simulink model "Urban_Air_Mobility_v3"  (R2021a)
settings: Solver=ode4  StartTime=0.0  StopTime=50  FixedStep=0.01  RelTol=1e-3
model workspace (MAT data in the model file):
  op_trim2 : handle (value not decoded)
undefined symbols (not defined in the file or in its folder): BackProp, Earth, ForwProp, geo, initialise, mass, simsetup, WGS84
libraries: dspindex x6, aerolibactuator x4, sharedutil x3, simulink x3, aerolibasang x2, aerolibtransform2 x2, aerolibutil x2, shared6dof x1, aerolibatmos2 x1, sharedtransform x1, aerolibconvert2 x1
(part 3 of 3)

== system Urban_Air_Mobility_v3/Urban Air Vehicle Airframe Flight Dynamic Model/Landing_gear_Model/Landing Gear (with steer 4)/Main_gear_right_friction_forces/Velocity at MGR in ground path ==
  DCM_B_to_E : Inport
  V_b : Inport  Port=2
  "[p, q, r]" : Inport  Port=3
  P_gear : Inport  Port=4
  P_cg : Inport  Port=5
  Euler : Inport  Port=6
  Demux : Demux  Outputs=3
  Ground Path Velocities : Subsystem
  Matrix Multiply1 : Product  Multiplication=Matrix(*)
  Mux2 : Mux  Inputs=3
  Velocity at gear in body axes : MATLAB Function  TreatAsAtomicUnit=on
  u_g_gp : Outport  VectorParamsAs1DForOutWhenUnconnected=off
  v_g_gp : Outport  Port=2  VectorParamsAs1DForOutWhenUnconnected=off
  wires:
  P_cg/1 -> Velocity at gear in body axes/6(P_cg)
  Ground Path Velocities/2(v_ng_ground_path) -> v_g_gp/1
  Euler/1 -> Ground Path Velocities/2("Euler ")
  Ground Path Velocities/1(u_ng_ground_path) -> u_g_gp/1
  "[p, q, r]"/1 -> Demux/1
  V_b/1 -> Velocity at gear in body axes/1(V_b)
  P_gear/1 -> Velocity at gear in body axes/5(P_g)
  Demux/2 -> Velocity at gear in body axes/3(q)
  Velocity at gear in body axes/3(w_g) -> Mux2/3
  Mux2/1 -> Matrix Multiply1/2  "[u_ng, v_ng, w_ng]_body"
  Velocity at gear in body axes/1(u_g) -> Mux2/1
  Matrix Multiply1/1 -> Ground Path Velocities/1(V_ng_earth)  "V_ng_earth"
  Velocity at gear in body axes/2(v_g) -> Mux2/2
  DCM_B_to_E/1 -> Matrix Multiply1/1
  Demux/3 -> Velocity at gear in body axes/4(r)
  Demux/1 -> Velocity at gear in body axes/2(p)

== system Urban_Air_Mobility_v3/Urban Air Vehicle Airframe Flight Dynamic Model/Landing_gear_Model/Landing Gear (with steer 4)/Nose_gear_friction_forces/GP to Earth axes  ==
  Euler Angles : Inport
  F_long_g : Inport  Port=2
  F_lat_g : Inport  Port=3
  nose_wheel_angle (rad) : Inport  Port=4
  Add : Sum
  Ground : Ground
  Multiply{9..12} (4 alike) : Product
  Selector6 : Selector  InputPortWidth=3  IndexOptions=Index vector (dialog)  Indices=3  OutputSizes=1
  Sin : Trigonometry
  Sin1 : Trigonometry  Operator=cos
  Subtract : Sum  Inputs=+-
  Subtract1 : Sum
  Terminator : Terminator
  Fx_g_E : Outport  VectorParamsAs1DForOutWhenUnconnected=off
  Fy_g_E : Outport  Port=2  VectorParamsAs1DForOutWhenUnconnected=off
  wires:
  [cos_psi] -> Multiply9/2
  Euler Angles/1 -> Selector6/1
  Multiply10/1 -> Subtract/2
  Sin/1 -> [sin_psi]
  Multiply12/1 -> Subtract1/1
  F_lat_g/1 -> Multiply11/1, Multiply10/2
  F_long_g/1 -> Multiply9/1, Multiply12/1
  Subtract1/1 -> Fy_g_E/1  "Fy_g_E"
  Subtract/1 -> Fx_g_E/1  "Fx_g_E"
  [sin_psi] -> Multiply10/1
  [sin_psi] -> Multiply12/2
  [cos_psi] -> Multiply11/2
  Multiply11/1 -> Subtract1/2
  Multiply9/1 -> Subtract/1
  Sin1/1 -> [cos_psi]
  Selector6/1 -> Add/1  "psi"
  nose_wheel_angle (rad)/1 -> Terminator/1
  Add/1 -> Sin1/1, Sin/1
  Ground/1 -> Add/2

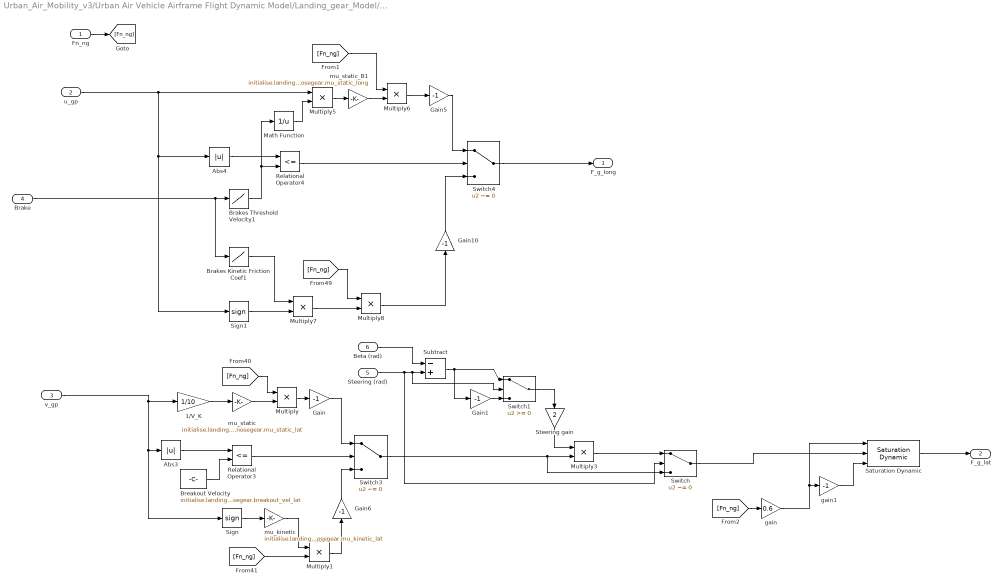
== system Urban_Air_Mobility_v3/Urban Air Vehicle Airframe Flight Dynamic Model/Landing_gear_Model/Landing Gear (with steer 4)/Nose_gear_friction_forces/NG_friction_forces ==
  "Fn_ng " : Inport
  u_gp : Inport  Port=2
  v_gp : Inport  Port=3
  Brake : Inport  Port=4
  "Steering (rad) " : Inport  Port=5
  "Beta (rad) " : Inport  Port=6
  1/V_K : Gain  Gain=1/10
  Abs3 : Abs
  Abs4 : Abs
  Brakes Kinetic Friction Coef1 : Lookup  InputValues=[0 1]  Table=[0.1 0.3]
  Brakes Threshold Velocity1 : Lookup  InputValues=[0 1]  Table=[0.5, 0.04]
  Breakout Velocity : Constant  Value=initialise.landinggear.nosegear.breakout_vel_lat
  Gain{,1,5..6,10} (5 alike) : Gain  Gain=-1
  Math Function : Math  Operator=reciprocal  SignedPower=on  SaturateOnIntegerOverflow=on
  Multiply{,1,3,5..8} (7 alike) : Product
  Relational Operator3 : RelationalOperator  Operator=<=  OutDataTypeStr=boolean  RndMeth=Simplest
  Relational Operator4 : RelationalOperator  Operator=<=  OutDataTypeStr=boolean  RndMeth=Simplest
  Saturation Dynamic : simulink/Discontinuities/Saturation Dynamic  OutMin=[]  OutMax=[]  OutDataTypeStr=Inherit: Same as second input  OutDataType=fixdt(1, 16)  OutScaling=2^-10  DoSatur=off
  Sign : Signum
  Sign1 : Signum
  Steering gain : Gain  Gain=2
  Subtract : Sum  Inputs=-+
  Switch : Switch  Criteria=u2 ~= 0
  Switch1 : Switch
  Switch3 : Switch  Criteria=u2 ~= 0
  Switch4 : Switch  Criteria=u2 ~= 0
  gain : Gain  Gain=0.6
  gain1 : Gain  Gain=-1
  mu_kinetic : Gain  Gain=initialise.landinggear.nosegear.mu_kinetic_lat
  mu_static : Gain  Gain=initialise.landinggear.nosegear.mu_static_lat
  mu_static_B1 : Gain  Gain=initialise.landinggear.nosegear.mu_static_long
  F_g_long : Outport  VectorParamsAs1DForOutWhenUnconnected=off
  F_g_lat : Outport  Port=2  VectorParamsAs1DForOutWhenUnconnected=off
  wires:
  Multiply1/1 -> Gain6/1
  Switch4/1 -> F_g_long/1
  Math Function/1 -> Multiply5/2
  Abs4/1 -> Relational Operator4/1
  Sign1/1 -> Multiply7/2
  Multiply5/1 -> mu_static_B1/1
  u_gp/1 -> Multiply5/1, Sign1/1, Abs4/1
  Multiply6/1 -> Gain5/1
  Brakes Threshold Velocity1/1 -> Relational Operator4/2, Math Function/1
  Multiply8/1 -> Gain10/1
  Multiply7/1 -> Multiply8/2
  [Fn_ng] -> Multiply8/1
  mu_static/1 -> Multiply/2
  Multiply/1 -> Gain/1
  Relational Operator4/1 -> Switch4/2
  Gain5/1 -> Switch4/1
  mu_static_B1/1 -> Multiply6/2
  v_gp/1 -> 1/V_K/1, Sign/1, Abs3/1
  mu_kinetic/1 -> Multiply1/1
  Gain10/1 -> Switch4/3
  Abs3/1 -> Relational Operator3/1
  [Fn_ng] -> Multiply/1
  Sign/1 -> mu_kinetic/1
  1/V_K/1 -> mu_static/1
  Relational Operator3/1 -> Switch3/2
  Gain/1 -> Switch3/1
  Breakout Velocity/1 -> Relational Operator3/2
  Brakes Kinetic Friction Coef1/1 -> Multiply7/1
  [Fn_ng] -> Multiply1/2
  Brake/1 -> Brakes Kinetic Friction Coef1/1, Brakes Threshold Velocity1/1
  Gain6/1 -> Switch3/3
  "Fn_ng "/1 -> [Fn_ng]
  [Fn_ng] -> Multiply6/1
  Switch3/1 -> Switch/3, Multiply3/2
  "Steering (rad) "/1 -> Switch/2, Switch1/2, Subtract/2
  Saturation Dynamic/1 -> F_g_lat/1
  [Fn_ng] -> gain/1
  gain/1 -> Saturation Dynamic/1, gain1/1
  gain1/1 -> Saturation Dynamic/3
  Multiply3/1 -> Switch/1
  Switch/1 -> Saturation Dynamic/2
  "Beta (rad) "/1 -> Subtract/1
  Subtract/1 -> Gain1/1, Switch1/1
  Gain1/1 -> Switch1/3
  Switch1/1 -> Steering gain/1
  Steering gain/1 -> Multiply3/1

== system Urban_Air_Mobility_v3/Urban Air Vehicle Airframe Flight Dynamic Model/Landing_gear_Model/Landing Gear (with steer 4)/Nose_gear_friction_forces/Velocity at NG in ground path ==
  DCM_B_to_E : Inport
  V_b : Inport  Port=2
  "[p, q, r]" : Inport  Port=3
  P_gear : Inport  Port=4
  P_cg : Inport  Port=5
  Euler : Inport  Port=6
  "nose_wheel_steering (rad) " : Inport  Port=7
  Demux : Demux  Outputs=3
  Ground Path Velocities : Subsystem
  Matrix Multiply1 : Product  Multiplication=Matrix(*)
  Mux2 : Mux  Inputs=3
  Scope : Scope
  Scope1 : Scope
  Velocity at gear in body axes : MATLAB Function  TreatAsAtomicUnit=on
  u_g_gp : Outport  VectorParamsAs1DForOutWhenUnconnected=off
  v_g_gp : Outport  Port=2  VectorParamsAs1DForOutWhenUnconnected=off
  wires:
  Demux/1 -> Velocity at gear in body axes/2(p)
  Demux/3 -> Velocity at gear in body axes/4(r)
  DCM_B_to_E/1 -> Matrix Multiply1/1
  Velocity at gear in body axes/2(v_g) -> Mux2/2
  Matrix Multiply1/1 -> Ground Path Velocities/1(V_ng_earth)  "V_ng_earth"
  Velocity at gear in body axes/1(u_g) -> Mux2/1
  Mux2/1 -> Matrix Multiply1/2  "[u_ng, v_ng, w_ng]_body"
  Velocity at gear in body axes/3(w_g) -> Mux2/3
  Demux/2 -> Velocity at gear in body axes/3(q)
  P_gear/1 -> Velocity at gear in body axes/5(P_g)
  V_b/1 -> Velocity at gear in body axes/1(V_b)
  "[p, q, r]"/1 -> Demux/1
  Ground Path Velocities/1(u_ng_ground_path) -> Scope/1, u_g_gp/1
  Euler/1 -> Ground Path Velocities/2("Euler ")
  Ground Path Velocities/2(v_ng_ground_path) -> Scope1/1, v_g_gp/1
  P_cg/1 -> Velocity at gear in body axes/6(P_cg)
  "nose_wheel_steering (rad) "/1 -> Ground Path Velocities/3(node_steer_angle (rad))

== system Urban_Air_Mobility_v3/Urban Air Vehicle Airframe Flight Dynamic Model/Landing_gear_Model/Landing Gear (with steer 4)/Main_gear_left_friction_forces/Velocity at MGL in ground path/Ground Path Velocities ==
  V_ng_earth : Inport
  "Euler " : Inport  Port=2
  Add : Sum
  Add3 : Sum
  Gain1 : Gain  Gain=-1
  Multiply{,1..3} (4 alike) : Product
  Scope : Scope
  Selector3 : Selector  InputPortWidth=3  IndexOptions=Index vector (dialog)  Indices=1  OutputSizes=1
  Selector4 : Selector  InputPortWidth=3  IndexOptions=Index vector (dialog)  Indices=2  OutputSizes=1
  Selector5 : Selector  InputPortWidth=3  IndexOptions=Index vector (dialog)  Indices=3  OutputSizes=1
  Sin : Trigonometry
  Sin1 : Trigonometry  Operator=cos
  u_ng_ground_path : Outport  VectorParamsAs1DForOutWhenUnconnected=off
  v_ng_ground_path : Outport  Port=2  VectorParamsAs1DForOutWhenUnconnected=off
  wires:
  V_ng_earth/1 -> Scope/1, Selector4/1, Selector3/1
  Add/1 -> u_ng_ground_path/1  "u_ng_ground_path"
  Selector4/1 -> Multiply2/2, Multiply1/2  "v_ng_earth"
  Multiply2/1 -> Add3/2
  Sin1/1 -> Multiply/2, Multiply2/1
  Sin/1 -> Multiply3/2, Multiply1/1
  Multiply/1 -> Add/1
  Selector3/1 -> Multiply3/1, Multiply/1  "u_ng_earth"
  Multiply1/1 -> Add/2
  Multiply3/1 -> Gain1/1
  Gain1/1 -> Add3/1
  "Euler "/1 -> Selector5/1
  Add3/1 -> v_ng_ground_path/1  "v_ng_ground_path"
  Selector5/1 -> Sin1/1, Sin/1  "psi"

== system Urban_Air_Mobility_v3/Urban Air Vehicle Airframe Flight Dynamic Model/Landing_gear_Model/Landing Gear (with steer 4)/Main_gear_right_friction_forces/Velocity at MGR in ground path/Ground Path Velocities ==
  V_ng_earth : Inport
  "Euler " : Inport  Port=2
  Add : Sum
  Add3 : Sum
  Gain1 : Gain  Gain=-1
  Multiply{,1..3} (4 alike) : Product
  Scope : Scope
  Selector3 : Selector  InputPortWidth=3  IndexOptions=Index vector (dialog)  Indices=1  OutputSizes=1
  Selector4 : Selector  InputPortWidth=3  IndexOptions=Index vector (dialog)  Indices=2  OutputSizes=1
  Selector5 : Selector  InputPortWidth=3  IndexOptions=Index vector (dialog)  Indices=3  OutputSizes=1
  Sin : Trigonometry
  Sin1 : Trigonometry  Operator=cos
  u_ng_ground_path : Outport  VectorParamsAs1DForOutWhenUnconnected=off
  v_ng_ground_path : Outport  Port=2  VectorParamsAs1DForOutWhenUnconnected=off
  wires:
  Add3/1 -> v_ng_ground_path/1  "v_ng_ground_path"
  "Euler "/1 -> Selector5/1
  Gain1/1 -> Add3/1
  Multiply3/1 -> Gain1/1
  Multiply1/1 -> Add/2
  Selector3/1 -> Multiply/1, Multiply3/1  "u_ng_earth"
  Multiply/1 -> Add/1
  Sin/1 -> Multiply1/1, Multiply3/2
  Sin1/1 -> Multiply2/1, Multiply/2
  Multiply2/1 -> Add3/2
  Selector4/1 -> Multiply1/2, Multiply2/2  "v_ng_earth"
  Add/1 -> u_ng_ground_path/1  "u_ng_ground_path"
  V_ng_earth/1 -> Selector3/1, Selector4/1, Scope/1
  Selector5/1 -> Sin1/1, Sin/1  "psi"

== system Urban_Air_Mobility_v3/Urban Air Vehicle Airframe Flight Dynamic Model/Landing_gear_Model/Landing Gear (with steer 4)/Nose_gear_friction_forces/Velocity at NG in ground path/Ground Path Velocities ==
  V_ng_earth : Inport
  "Euler " : Inport  Port=2
  node_steer_angle (rad) : Inport  Port=3
  Add : Sum
  Add1 : Sum
  Add3 : Sum
  Gain1 : Gain  Gain=-1
  Multiply{,1..3} (4 alike) : Product
  Scope : Scope
  Selector3 : Selector  InputPortWidth=3  IndexOptions=Index vector (dialog)  Indices=1  OutputSizes=1
  Selector4 : Selector  InputPortWidth=3  IndexOptions=Index vector (dialog)  Indices=2  OutputSizes=1
  Selector5 : Selector  InputPortWidth=3  IndexOptions=Index vector (dialog)  Indices=3  OutputSizes=1
  Sin : Trigonometry
  Sin1 : Trigonometry  Operator=cos
  u_ng_ground_path : Outport  VectorParamsAs1DForOutWhenUnconnected=off
  v_ng_ground_path : Outport  Port=2  VectorParamsAs1DForOutWhenUnconnected=off
  wires:
  V_ng_earth/1 -> Scope/1, Selector4/1, Selector3/1
  Add/1 -> u_ng_ground_path/1  "u_ng_ground_path"
  Selector4/1 -> Multiply2/2, Multiply1/2  "v_ng_earth"
  Multiply2/1 -> Add3/2
  Sin1/1 -> Multiply/2, Multiply2/1
  Sin/1 -> Multiply3/2, Multiply1/1
  Multiply/1 -> Add/1
  Selector3/1 -> Multiply3/1, Multiply/1  "u_ng_earth"
  Multiply1/1 -> Add/2
  Multiply3/1 -> Gain1/1
  Gain1/1 -> Add3/1
  "Euler "/1 -> Selector5/1
  Add3/1 -> v_ng_ground_path/1  "v_ng_ground_path"
  Selector5/1 -> Add1/1  "psi"
  node_steer_angle (rad)/1 -> Add1/2
  Add1/1 -> Sin/1, Sin1/1

== matlab function Urban_Air_Mobility_v3/Urban Air Vehicle Airframe Flight Dynamic Model/Back propeller/MATLAB Function ==
  data: UVW input; TAS_prop output; PQR input; prop_pos input; alpha_prop output; beta_prop output; DCM_prop2b output
function [TAS_prop,alpha_prop,beta_prop,DCM_prop2b] = fcn(UVW,PQR,prop_pos)
%Initialize vectors
UVW = [UVW(1) UVW(2) UVW(3)];
% UVW = [-UVW(3) UVW(2) UVW(1)];%what it would like on that position, used
% b2prop axis matrix transformation instead
PQR = [PQR(1) PQR(2) PQR(3)];
prop_pos = [prop_pos(1) prop_pos(2) prop_pos(3)];

DCM_b2prop = [0 0 -1;
              0 1 0;
              1 0 0];
%UVW calculation v = v0 + w^r (rigid body)
WR_ba = cross(PQR,prop_pos);
UVW_prop = (DCM_b2prop*UVW')' + (DCM_b2prop*cross(PQR,prop_pos)')';

%outputs
TAS_prop = norm(UVW_prop);

if TAS_prop < 10
    alpha_prop = 0;
    beta_prop = 0;
else
    alpha_prop = atan(UVW_prop(3)/UVW_prop(1));
    beta_prop = asin(UVW_prop(2)/TAS_prop);
end
DCM_prop2b = [0 0 1;
        0 1 0;
        -1 0 0];
end

== matlab function Urban_Air_Mobility_v3/Urban Air Vehicle Airframe Flight Dynamic Model/Equations of motion/Incidence, Sideslip, & Airspeed2 ==
  data: V_body input; alpha output; beta output; VTAS output
function [alpha,beta,VTAS] = fcn(V_body)
u=V_body(1);
v=V_body(2);
w=V_body(3);
if u==0 & v==0 & w==0
    alpha=0;
    beta=0;
    VTAS=0;
else
     alpha=atan2(w,u);
    VTAS=sqrt(u*u+v*v+w*w);
    if VTAS~=0
        beta=asin(v/VTAS);
    else
        beta=0;
    end
    
end





return

== matlab function Urban_Air_Mobility_v3/Urban Air Vehicle Airframe Flight Dynamic Model/Forward Right propeller/Propeller Function ==
  data: V input; Forces output; n input; alpha input; beta input; density input; Sn input; Ap input; pitch075 input; J_Table input; CP_Table input; CT_Table input; prop_type input; sigma_e input; Power output; e_p output; TC output; D input
function [Forces,Power,e_p,TC] = prop_model(V,n, alpha,beta,density,Sn,Ap,pitch075,...
                           J_Table,CP_Table,CT_Table,prop_type,sigma_e,D)
%prop_model: Propeller power and forces calculation in the spinner axis. 
% Method based on strip theory which was applicable to small or moderate
% inclination angles (approx. <20deg). The method also calculates the prop
% downwash caused by the slipstream.
% V:        Airspeed (m/s)
% n:        Rotor speed (rps) (<0 if prop rotates clockwise)
% alpha: 	Rotor angle of attack (rad)
% beta:     Rotor sideslip (rad)
% density:  Air density
%
% Sn:       Nacelle area
% Ap        prop disk area
% pitch075:    Prop pitch angle referred to zero-lift line of section 0.75R (deg)
% J_Table:  Table of advance ratio
% CP_Table: Table of CP
% CT_Table: Table of CT
% prop_type: 1 single prop, 2 coaxial prop
% sigma_e:  Propeller solidity

if n ~= 0
    % advance ratio
    J = V /(abs(n)* D);
else
    J = 0;
end
% corrected advance ratio
% ESDU86017
Jeff = J * (1 - 0.255*Sn/Ap);

% propeller CP
CP = interp1(J_Table,CP_Table,Jeff,'linear','extrap');      
% propeller CT
CT = interp1(J_Table,CT_Table,Jeff,'linear','extrap');

if J ~= 0
    % ESDU 89047 
    Tc = CT * 8/(pi * J^2);
    kb = tan(pi/180*(pitch075 - 5))/(sigma_e * cos(pi/180*(pitch075 - 5)));
    if prop_type == 1
        CZ_alpha = -((4.25 * sigma_e)/(1 + 2 * sigma_e)) * sin(pi/180*(pitch075 + 3))*...
            (1 + ((3 * Tc/8)/sqrt(1 + (2*Tc/3))));  
        Cn_CZ = -(0.321/(sigma_e + tan(pi/180*(pitch075 + 5)))) * (1 + ((Tc * kb/3)...
            /(1 + (3 * Tc * sqrt(kb)/4))));
        CZ_alpha = CZ_alpha * (CT/Tc); 
        Cn_alpha = Cn_CZ * CZ_alpha;
    else
        CZ_alpha = -((3.86 * sigma_e)/(1 + sigma_e)) * sin(pi/180*(pitch075 + 9))*...
            (1 + ((3 * Tc/8)/sqrt(1 + (2*Tc/3))));
        CZ_alpha = CZ_alpha * (CT/Tc);   
        Cn_alpha = 0;
    end
else
    Tc=0;
    
    CZ_alpha =0;
    Cn_alpha =0;
end
Forces = zeros(6,1); 

%CT>0
% correction based on ESDU86017 for nacelle effect
Forces(1) = density*n^2*D^4*CT*(1 - 0.255*Sn/Ap);
% CY_beta sign of n (<0 if clockwise) 
Forces(2) = -sign(n)*density*n^2*D^4*CZ_alpha*beta;
% CZ_apha < 0 
Forces(3) = density*n^2*D^4*CZ_alpha*alpha;
Forces(4) = density*n^2*D^5*CP/(2*pi);
% Cm_beta sign of n (<0 if clockwise) 
Forces(5) = sign(n)*density*n^2*D^5*Cn_alpha*beta;
% Cn_alpha - sign of n (>0 if clockwise) 
Forces(6) = - sign(n)*density*n^2*D^5*Cn_alpha*beta;
       
Power = density*n^3*D^5*CP;

% Downwash caused by propeller slipstream based on LabanOn-line Aircraft
% Aerodynamic Model Identification. PhD thesis, Proefschrift Technische
% Universiteit Delft, 1994.
e_p = (Forces(1)*sin(alpha)-Forces(3)*cos(alpha))/(density*V^2*Ap);
TC = Tc*pi/8;

end

== matlab function Urban_Air_Mobility_v3/Urban Air Vehicle Airframe Flight Dynamic Model/Forces and Moments calculation/Calculate aero coefficients ==
  data: forces input; CForces output; moments input; geo input; q_dyn input; CMoments output
function [CForces,CMoments] = fcn(forces,moments,geo,q_dyn)

if q_dyn <= 0
    CForces = [0 0 0]';
    CMoments = [0 0 0]';

else
    CForces = forces./(q_dyn*geo(1));
    X = [q_dyn*(geo(1)*geo(3)); q_dyn*(geo(1)*geo(2)); q_dyn*(geo(1)*geo(3))];
    CMoments = moments./X;
end

return

== matlab function Urban_Air_Mobility_v3/Urban Air Vehicle Airframe Flight Dynamic Model/Forces and Moments calculation/Ground Effect /MATLAB Function1 ==
  data: lift_curve_slope input; height_above_ground input; delta_CL output; c_bar input; b input; AR input; Drag input; Lift input; CL_dF input; Cm_dF input; Flap input; wing_thickness input; delta_CD output; q_dyn input; S_ref input; delta_Lift output; delta_Drag output; VTAS input
function [delta_CL, delta_CD, delta_Lift, delta_Drag ] = Ground_effect(lift_curve_slope, height_above_ground,c_bar, b, AR, Drag, Lift, CL_dF, Cm_dF, Flap, wing_thickness, q_dyn, S_ref, VTAS)
% Equations taken from ESDU 72023:

if (VTAS<=5)
    delta_CL=0;
    delta_CD=0;
    delta_Lift=0;
    delta_Drag=0;
else
    
    CL=Lift/(q_dyn*S_ref);
    CD=Drag/(q_dyn*S_ref);

    Cm_F=Cm_dF*Flap;
    CL_F=CL_dF*Flap;

    %LIFT:
    h=height_above_ground; %height above ground of quarter chord point of aero. mean chord of wing.
    A=AR; %=b/c_bar or =b^2/S
    t=wing_thickness; %max thickness/chord ratio of wing
    a=lift_curve_slope;

    r=sqrt(1+(2*h/b)^2)-2*h/b;
    sigma=exp(-2.48*(2*h/b)^0.768);
    tau=(h/c_bar)/(8*pi*(h/c_bar)^2+1/64);
    N_prime=1+0.00239*(10*(c_bar/h)+16*(c_bar/h)^2+(c_bar/h)^3); %??
    % if(isfinite(N_prime))
    %     N=1+(N_prime-1)*(1+2/CL*Cm_dF);
    % else
    %     N_prime=1;
    %     N=1+(N_prime-1)*(1+2/CL*Cm_dF);
    % end
    N=1+(N_prime-1)*(1+2/CL*Cm_F);
    c1=a*sigma/(pi*A);
    delta_CL= CL/(1-c1)*(c1+r*(N/(1+tau*N*CL/(1-c1))^2-1));

    if(CL<0.7)
        delta_CL_t0=-0.165*t^1.5/(h/c_bar)^2.5;
        delta_CL_t=r*(1-1.4*CL)*delta_CL_t0;
    else
        delta_CL_t=0;
    end
    % if(isfinite(delta_CL_t))
    %     
    % else
    %     delta_CL_t=0;
    % end

    delta_CL=delta_CL + delta_CL_t;
    delta_Lift= delta_CL*q_dyn*S_ref;

    %DRAG:
    delta_CL_HLD=CL_F; %increment in lift due to high lift devices
    K=0.13; %function for vortex drag due to flaps (ESDU Aero F.02.01.08)
    one_plus_delta=1.01; %(1+delta)=vortex drag factor due to wing trailing vortices (ESDU 74035 or 01007).

    CD_v=(one_plus_delta)*CL^2/(pi*A)+K^2*(delta_CL_HLD)^2; 
    phi=0.00066*(570*b/h-32*(b/h)^2+(b/h)^3);
    % if(isfinite(phi))
    %     
    % else
    %     phi=0;
    % end

    delta_CD=-phi*CL/(pi*A)*CD-(sigma-(2-sigma)*phi*CL/(pi*A))*CD_v;
    delta_Drag= delta_CD*q_dyn*S_ref;
end

== matlab function Urban_Air_Mobility_v3/Urban Air Vehicle Airframe Flight Dynamic Model/Forces and Moments calculation/Aerodynamics ==
  data: Drag output; Sideforce output; Trim input; Lift output; LatDir input; Long input; Control input; states input; inputs input; geo input; dyn_pres input; V input; Rolling output; Pitching output; Yawing output; UC_forces input; K input
function [Drag,Sideforce,Lift,Rolling,Pitching,Yawing] = fcn(Trim,LatDir,Long,Control,states,inputs,geo,dyn_pres,V,UC_forces,K)

% states = [alpha beta p q r]
% inputs = [InnerAil OuterAil RightRudder LeftRudder]
% geo = [Sref Cref Bref]

%Parameter declaration
%states
alpha = states(1);
beta = states(2);
p = states(3);
q = states(4);
r = states(5);
%inputs
inA = inputs(1);
outA = inputs(2);
Rr = inputs(3);
Rl = inputs(4);
%Reference magnitudes
Sref = geo(1);
Cref = geo(2);
Bref = geo(3);
%Trim conditions
CL_0 = Trim(1);
CD_0 = Trim(2);
Cm_0 = Trim(3);
%Longitudinal derivatives
CL_alpha = Long(1);
CL_q = Long(2);
Cm_alpha = Long(3);
Cm_q = Long(4);
%Lateral-Directional derivatives
Cn_p = LatDir(1);
Cn_r = LatDir(2);
Cl_p = LatDir(3);
Cl_r = LatDir(4);
CY_p = LatDir(5);
CY_r = LatDir(6);
CY_b = LatDir(7);
Cl_b = LatDir(8);
Cn_b = LatDir(9);
%Control derivatives
CL_dinA = Control(1);
Cm_dinA = Control(2);
CD_dinA = Control(3);
CY_doutA = Control(4);
Cl_doutA = Control(5);
Cn_doutA = Control(6);
CD_doutA = Control(7);
CY_dRr = Control(8);
Cl_dRr = Control(9);
Cn_dRr = Control(10);
CD_dRr = Control(11);
CY_dRl = Control(12);
Cl_dRl = Control(13);
Cn_dRl = Control(14);
CD_dRl = Control(15);
%Undercarriage forces and moments
L_UC = 0;
D_UC = 0;
Y_UC = 0;
l_UC = 0;
m_UC = 0;
n_UC = 0;

%Coefficient 
K = K;%Oswald factor


if V <= 5
    Lift = 0;
    Drag = 0;
    Sideforce = 0;
    Rolling = 0;
    Pitching = 0;
    Yawing = 0;
    
else
    
    Lift = dyn_pres*Sref*(CL_0+CL_alpha*alpha+CL_q*q*Cref/(2*V)+...
        + CL_dinA*inA) +L_UC;
    
    Drag = dyn_pres*Sref*(CD_0+K*(Lift/(dyn_pres*Sref))^2+CD_dinA*inA...
        +CD_doutA*outA+CD_dRr*Rr+CD_dRl*Rl)+ D_UC;
    
    Sideforce = dyn_pres*Sref*(CY_b*beta+CY_p*p*Bref/(2*V)+CY_r*r*Bref/(2*V)...
        +CY_doutA*outA+CY_dRr*Rr+CY_dRl*Rl)+ Y_UC;
    
    Rolling = dyn_pres*Sref*Bref*(Cl_b*beta+Cl_p*p*Bref/(2*V)...
        +Cl_r*r*Bref/(2*V)+Cl_doutA*outA+Cl_dRr*Rr+Cl_dRl*Rl)+ l_UC;
    
    Pitching = dyn_pres*Sref*Cref*(Cm_0+Cm_alpha*alpha+Cm_q*q*Cref/(2*V)...
        + Cm_dinA*inA) + m_UC;
    
    Yawing = dyn_pres*Sref*Bref*(Cn_b*beta*Cn_p*p*Bref/(2*V)+Cn_r*r*Bref/(2*V)+...
       +Cn_doutA*outA+Cn_dRr*Rr+Cn_dRl*Rl)+ n_UC;
   
end


return

== matlab function Urban_Air_Mobility_v3/Urban Air Vehicle Airframe Flight Dynamic Model/Landing_gear_Model/Landing Gear (with steer 4)/Main_gear_left_friction_forces/Velocity at MGL in ground path/Velocity at gear in body axes ==
  data: V_b input; u_g output; p input; q input; r input; P_g input; P_cg input; v_g output; w_g output
function [u_g, v_g, w_g] = fcn(V_b, p, q, r, P_g, P_cg)

u=V_b(1);
v=V_b(2);
w=V_b(3);

x_g=P_g(1);
y_g=P_g(2);
z_g=P_g(3);

x_cg=P_cg(1);
y_cg=P_cg(2);
z_cg=P_cg(3);


u_g= u+ q*(z_g-z_cg) - r*(y_g - y_cg);
v_g= v+ r*(x_g-x_cg) - p*(z_g - z_cg);
w_g= w+ p*(y_g-y_cg) - q*(x_g - x_cg);

== matlab function Urban_Air_Mobility_v3/Urban Air Vehicle Airframe Flight Dynamic Model/Landing_gear_Model/Landing Gear (with steer 4)/Main_gear_right_friction_forces/Velocity at MGR in ground path/Velocity at gear in body axes ==
  data: V_b input; u_g output; p input; q input; r input; P_g input; P_cg input; v_g output; w_g output
function [u_g, v_g, w_g] = fcn(V_b, p, q, r, P_g, P_cg)

u=V_b(1);
v=V_b(2);
w=V_b(3);

x_g=P_g(1);
y_g=P_g(2);
z_g=P_g(3);

x_cg=P_cg(1);
y_cg=P_cg(2);
z_cg=P_cg(3);


u_g= u+ q*(z_g-z_cg) - r*(y_g - y_cg);
v_g= v+ r*(x_g-x_cg) - p*(z_g - z_cg);
w_g= w+ p*(y_g-y_cg) - q*(x_g - x_cg);

== matlab function Urban_Air_Mobility_v3/Urban Air Vehicle Airframe Flight Dynamic Model/Back propeller/Propeller Function ==
  data: V input; Forces output; n input; alpha input; beta input; density input; Sn input; Ap input; pitch075 input; J_Table input; CP_Table input; CT_Table input; prop_type input; sigma_e input; Power output; e_p output; TC output; D input
function [Forces,Power,e_p,TC] = prop_model(V,n, alpha,beta,density,Sn,Ap,pitch075,...
                           J_Table,CP_Table,CT_Table,prop_type,sigma_e,D)
%prop_model: Propeller power and forces calculation in the spinner axis. 
% Method based on strip theory which was applicable to small or moderate
% inclination angles (approx. <20deg). The method also calculates the prop
% downwash caused by the slipstream.
% V:        Airspeed (m/s)
% n:        Rotor speed (rps) (<0 if prop rotates clockwise)
% alpha: 	Rotor angle of attack (rad)
% beta:     Rotor sideslip (rad)
% density:  Air density
%
% Sn:       Nacelle area
% Ap        prop disk area
% pitch075:    Prop pitch angle referred to zero-lift line of section 0.75R (deg)
% J_Table:  Table of advance ratio
% CP_Table: Table of CP
% CT_Table: Table of CT
% prop_type: 1 single prop, 2 coaxial prop
% sigma_e:  Propeller solidity

if n ~= 0
    % advance ratio
    J = V /(abs(n)* D);
else
    J = 0;
end
% corrected advance ratio
% ESDU86017
Jeff = J * (1 - 0.255*Sn/Ap);

% propeller CP
CP = interp1(J_Table,CP_Table,Jeff,'linear','extrap');      
% propeller CT
CT = interp1(J_Table,CT_Table,Jeff,'linear','extrap');

if J ~= 0
    % ESDU 89047 
    Tc = CT * 8/(pi * J^2);
    kb = tan(pi/180*(pitch075 - 5))/(sigma_e * cos(pi/180*(pitch075 - 5)));
    if prop_type == 1
        CZ_alpha = -((4.25 * sigma_e)/(1 + 2 * sigma_e)) * sin(pi/180*(pitch075 + 3))*...
            (1 + ((3 * Tc/8)/sqrt(1 + (2*Tc/3))));  
        Cn_CZ = -(0.321/(sigma_e + tan(pi/180*(pitch075 + 5)))) * (1 + ((Tc * kb/3)...
            /(1 + (3 * Tc * sqrt(kb)/4))));
        CZ_alpha = CZ_alpha * (CT/Tc); 
        Cn_alpha = Cn_CZ * CZ_alpha;
    else
        CZ_alpha = -((3.86 * sigma_e)/(1 + sigma_e)) * sin(pi/180*(pitch075 + 9))*...
            (1 + ((3 * Tc/8)/sqrt(1 + (2*Tc/3))));
        CZ_alpha = CZ_alpha * (CT/Tc);   
        Cn_alpha = 0;
    end
else
    Tc=0;
    
    CZ_alpha =0;
    Cn_alpha =0;
end
Forces = zeros(6,1); 

%CT>0
% correction based on ESDU86017 for nacelle effect
Forces(1) = density*n^2*D^4*CT*(1 - 0.255*Sn/Ap);
% CY_beta sign of n (<0 if clockwise) 
Forces(2) = -sign(n)*density*n^2*D^4*CZ_alpha*beta;
% CZ_apha < 0 
Forces(3) = density*n^2*D^4*CZ_alpha*alpha;
Forces(4) = density*n^2*D^5*CP/(2*pi);
% Cm_beta sign of n (<0 if clockwise) 
Forces(5) = sign(n)*density*n^2*D^5*Cn_alpha*beta;
% Cn_alpha - sign of n (>0 if clockwise) 
Forces(6) = - sign(n)*density*n^2*D^5*Cn_alpha*beta;
       
Power = density*n^3*D^5*CP;

% Downwash caused by propeller slipstream based on LabanOn-line Aircraft
% Aerodynamic Model Identification. PhD thesis, Proefschrift Technische
% Universiteit Delft, 1994.
e_p = (Forces(1)*sin(alpha)-Forces(3)*cos(alpha))/(density*V^2*Ap);
TC = Tc*pi/8;

if V>40
    Forces = zeros(6,1); 
end
    
   
end

== matlab function Urban_Air_Mobility_v3/Urban Air Vehicle Airframe Flight Dynamic Model/Landing_gear_Model/Landing Gear (with steer 4)/Moments about CG ==
  data: P_ng input; L output size=1; P_mgr input; P_mgl input; F_ng input; F_mgr input; F_mgl input; M output size=1; N output size=1
function [L, M, N] = fcn( P_ng, P_mgr, P_mgl, F_ng, F_mgr, F_mgl)

x_ng=abs(P_ng(1));
y_ng=abs(P_ng(2));
z_ng=abs(P_ng(3));

x_mgr=abs(P_mgr(1));
y_mgr=abs(P_mgr(2));
z_mgr=abs(P_mgr(3));

x_mgl=abs(P_mgl(1));
y_mgl=abs(P_mgl(2));
z_mgl=abs(P_mgl(3));

Fx_ng=F_ng(1);
Fy_ng=F_ng(2);
Fz_ng=F_ng(3);

Fx_mgr=F_mgr(1);
Fy_mgr=F_mgr(2);
Fz_mgr=F_mgr(3);

Fx_mgl=F_mgl(1);
Fy_mgl=F_mgl(2);
Fz_mgl=F_mgl(3);

%Moments:
L= Fz_mgr*y_mgr - Fz_mgl*y_mgl - Fy_ng*z_ng - Fy_mgl*z_mgl - Fy_mgr*z_mgr; %Assuming y_ng=0;
M= -Fz_ng*x_ng + Fz_mgl*x_mgl + Fz_mgr*x_mgr;% + Fx_ng*z_ng + Fx_mgl*z_mgl + Fx_mgr*z_mgr;
N= Fy_ng*x_ng - Fy_mgr*x_mgr - Fy_mgl*x_mgl - Fx_mgr*y_mgr +Fx_mgl*y_mgl; %Assuming no steering! and y_ng=0;

== matlab function Urban_Air_Mobility_v3/Urban Air Vehicle Airframe Flight Dynamic Model/Landing_gear_Model/Landing Gear (with steer 4)/Nose_gear_friction_forces/Velocity at NG in ground path/Velocity at gear in body axes ==
  data: V_b input; u_g output; p input; q input; r input; P_g input; P_cg input; v_g output; w_g output
function [u_g, v_g, w_g] = fcn(V_b, p, q, r, P_g, P_cg)

u=V_b(1);
v=V_b(2);
w=V_b(3);

x_g=P_g(1);
y_g=P_g(2);
z_g=P_g(3);

x_cg=P_cg(1);
y_cg=P_cg(2);
z_cg=P_cg(3);


u_g= u+ q*(z_g-z_cg) - r*(y_g - y_cg);
v_g= v+ r*(x_g-x_cg) - p*(z_g - z_cg);
w_g= w+ p*(y_g-y_cg) - q*(x_g - x_cg);

== matlab function Urban_Air_Mobility_v3/Urban Air Vehicle Airframe Flight Dynamic Model/Landing_gear_Model/UC Aero Forces and Moments/MATLAB Function ==
  data: q_dyn input; UC_forces output; alpha input; beta input; CD_mg input; CD_ng input; dfy_mg input; dfy_ng input; z_mg input; z_ng input; UC_pos input
function UC_forces   = UC_forces( q_dyn, alpha, beta, CD_mg, CD_ng, dfy_mg, dfy_ng, z_mg, z_ng, UC_pos)
% Calculate the aero forces and moment in the body axes of the under
% carriage
F_mg = zeros(3,1);
F_ng = zeros(3,1);
UC_forces = zeros(6,1);

q_x = q_dyn*cos(beta)^2;
q_y = q_dyn*sin(beta)^2*sign(beta);

F_mg(1) = q_x*cos(alpha)*CD_mg;
F_mg(2) = q_y*dfy_mg;
F_mg(3) = q_x*sin(alpha)*CD_mg;

F_ng(1) = q_x*cos(alpha)*CD_ng;
F_ng(2) = q_y*dfy_ng;
F_ng(3) = q_x*sin(alpha)*CD_ng;

UC_pos(1,3) = z_mg;
UC_pos(2,3) = z_mg;
UC_pos(3,3) = z_ng;

M_mg1 = cross(UC_pos(1,:)',F_mg);
M_mg2 = cross(UC_pos(2,:)',F_mg);
M_ng = cross(UC_pos(3,:)',F_ng);

UC_forces(1:3) = 2*F_mg + F_ng;
UC_forces(4:6) = M_mg1 + M_mg2 + M_ng;

% fx = UC_forces(1);
% fy = UC_forces(2);
% fz = UC_forces(3);
% mx = UC_forces(4); 
% my = UC_forces(5);
% mz = UC_forces(6);
end

== matlab function Urban_Air_Mobility_v3/Urban Air Vehicle Airframe Flight Dynamic Model/Forward Left propeller/MATLAB Function ==
  data: UVW input; TAS_prop output; PQR input; prop_pos input; tilt_prop input; alpha_prop output; beta_prop output; DCM_prop2b output
function [TAS_prop,alpha_prop,beta_prop,DCM_prop2b] = fcn(UVW,PQR,prop_pos,tilt_prop)
%Initialize vectors
UVW = [UVW(1) UVW(2) UVW(3)];
PQR = [PQR(1) PQR(2) PQR(3)];
prop_pos = [prop_pos(1) prop_pos(2) prop_pos(3)];

%UVW calculation v = v0 + w^r (rigid body) 
UVW_prop = UVW + cross(PQR,prop_pos);

%outputs
TAS_prop = norm(UVW_prop);


if TAS_prop<10
    alpha_prop=0;
    beta_prop=0;
else
    alpha_prop = tilt_prop + atan(UVW_prop(3)/UVW_prop(1));
    beta_prop = asin(UVW_prop(2)/TAS_prop);
end

DCM_prop2b = [cos(tilt_prop) 0 sin(tilt_prop);
        0 1 0;
        -sin(tilt_prop) 0 cos(tilt_prop)];
    
end

== matlab function Urban_Air_Mobility_v3/Urban Air Vehicle Airframe Flight Dynamic Model/Forward Right propeller/Conversion to propeller axes ==
  data: UVW input; TAS_prop output; PQR input; prop_pos input; tilt_prop input; alpha_prop output; beta_prop output; DCM_prop2b output
function [TAS_prop,alpha_prop,beta_prop,DCM_prop2b] = fcn(UVW,PQR,prop_pos,tilt_prop)
%Initialize vectors
UVW = [UVW(1) UVW(2) UVW(3)];
PQR = [PQR(1) PQR(2) PQR(3)];
prop_pos = [prop_pos(1) prop_pos(2) prop_pos(3)];

%UVW calculation v = v0 + w^r (rigid body) 
UVW_prop = UVW + cross(PQR,prop_pos);

%outputs
TAS_prop = norm(UVW_prop);


if TAS_prop<10
    alpha_prop=0;
    beta_prop=0;
else
    alpha_prop = tilt_prop + atan(UVW_prop(3)/UVW_prop(1));
    beta_prop = asin(UVW_prop(2)/TAS_prop);
end

DCM_prop2b = [cos(tilt_prop) 0 sin(tilt_prop);
        0 1 0;
        -sin(tilt_prop) 0 cos(tilt_prop)];
    
end

== matlab function Urban_Air_Mobility_v3/Urban Air Vehicle Airframe Flight Dynamic Model/Forward Left propeller/Propeller Function ==
  data: V input; Forces output; n input; alpha input; beta input; density input; Sn input; Ap input; pitch075 input; J_Table input; CP_Table input; CT_Table input; prop_type input; sigma_e input; Power output; e_p output; TC output; D input
function [Forces,Power,e_p,TC] = prop_model(V,n, alpha,beta,density,Sn,Ap,pitch075,...
                           J_Table,CP_Table,CT_Table,prop_type,sigma_e,D)
%prop_model: Propeller power and forces calculation in the spinner axis. 
% Method based on strip theory which was applicable to small or moderate
% inclination angles (approx. <20deg). The method also calculates the prop
% downwash caused by the slipstream.
% V:        Airspeed (m/s)
% n:        Rotor speed (rps) (<0 if prop rotates clockwise)
% alpha: 	Rotor angle of attack (rad)
% beta:     Rotor sideslip (rad)
% density:  Air density
%
% Sn:       Nacelle area
% Ap        prop disk area
% pitch075:    Prop pitch angle referred to zero-lift line of section 0.75R (deg)
% J_Table:  Table of advance ratio
% CP_Table: Table of CP
% CT_Table: Table of CT
% prop_type: 1 single prop, 2 coaxial prop
% sigma_e:  Propeller solidity

if n ~= 0
    % advance ratio
    J = V /(abs(n)* D);
else
    J = 0;
end
% corrected advance ratio
% ESDU86017
Jeff = J * (1 - 0.255*Sn/Ap);

% propeller CP
CP = interp1(J_Table,CP_Table,Jeff,'linear','extrap');      
% propeller CT
CT = interp1(J_Table,CT_Table,Jeff,'linear','extrap');

if J ~= 0
    % ESDU 89047 
    Tc = CT * 8/(pi * J^2);
    kb = tan(pi/180*(pitch075 - 5))/(sigma_e * cos(pi/180*(pitch075 - 5)));
    if prop_type == 1
        CZ_alpha = -((4.25 * sigma_e)/(1 + 2 * sigma_e)) * sin(pi/180*(pitch075 + 3))*...
            (1 + ((3 * Tc/8)/sqrt(1 + (2*Tc/3))));  
        Cn_CZ = -(0.321/(sigma_e + tan(pi/180*(pitch075 + 5)))) * (1 + ((Tc * kb/3)...
            /(1 + (3 * Tc * sqrt(kb)/4))));
        CZ_alpha = CZ_alpha * (CT/Tc); 
        Cn_alpha = Cn_CZ * CZ_alpha;
    else
        CZ_alpha = -((3.86 * sigma_e)/(1 + sigma_e)) * sin(pi/180*(pitch075 + 9))*...
            (1 + ((3 * Tc/8)/sqrt(1 + (2*Tc/3))));
        CZ_alpha = CZ_alpha * (CT/Tc);   
        Cn_alpha = 0;
    end
else
    Tc=0;
    
    CZ_alpha =0;
    Cn_alpha =0;
end
Forces = zeros(6,1); 

%CT>0
% correction based on ESDU86017 for nacelle effect
Forces(1) = density*n^2*D^4*CT*(1 - 0.255*Sn/Ap);
% CY_beta sign of n (<0 if clockwise) 
Forces(2) = -sign(n)*density*n^2*D^4*CZ_alpha*beta;
% CZ_apha < 0 
Forces(3) = density*n^2*D^4*CZ_alpha*alpha;
Forces(4) = density*n^2*D^5*CP/(2*pi);
% Cm_beta sign of n (<0 if clockwise) 
Forces(5) = sign(n)*density*n^2*D^5*Cn_alpha*beta;
% Cn_alpha - sign of n (>0 if clockwise) 
Forces(6) = - sign(n)*density*n^2*D^5*Cn_alpha*beta;
       
Power = density*n^3*D^5*CP;

% Downwash caused by propeller slipstream based on LabanOn-line Aircraft
% Aerodynamic Model Identification. PhD thesis, Proefschrift Technische
% Universiteit Delft, 1994.
e_p = (Forces(1)*sin(alpha)-Forces(3)*cos(alpha))/(density*V^2*Ap);
TC = Tc*pi/8;


end
